simulink model "AMCLIB_TrackObsrv_BAM"  (Simulink 9.3)
settings: Solver=VariableStepAuto  StartTime=0.0  StopTime=10.0  RelTol=1e-3
settings Model: Creator=nxa18952  LastModifiedBy=nxa18952
settings DataIOCC: SaveFormat=Dataset  SignalLoggingSaveFormat=Dataset  ReturnWorkspaceOutputs=on
settings OptimizationCC: LifeSpan=auto
settings DebuggingCC: UnderspecifiedInitializationDetection=Simplified  MergeDetectMultiDrivingBlocksExec=error  FcnCallInpInsideContextMsg=error  SFUnexpectedBacktrackingDiag=error  SFNoUnconditionalDefaultTransitionDiag=error  SFExecutionAtInitializationDiag=warning  ArithmeticOperatorsInVariantConditions=error
settings HardwareCC: ProdBitPerPointer=64  ProdBitPerSizeT=64  ProdBitPerPtrDiffT=64  ProdLargestAtomicFloat=Float  ProdIntDivRoundTo=Zero  ProdEndianess=LittleEndian  ProdWordSize=64  ProdHWDeviceType=Intel->x86-64 (Windows64)
settings ModelReferenceCC: PropagateSignalLabelsOutOfModel=on
settings SFSimCC: SimUseLocalCustomCode=on
settings RTWCC: RTWUseLocalCustomCode=on
settings CodeAppCC: StateflowObjectComments=off
settings GRTTargetCC: TargetLangStandard=C99 (ISO)  CombineOutputUpdateFcns=on  GRTInterface=off
settings ConfigComp: CovMetricSettings=dwe  CovHtmlReporting=off  CovSaveCumulativeToWorkspaceVar=off  CovSaveSingleToWorkspaceVar=off  CovExternalEMLEnable=on

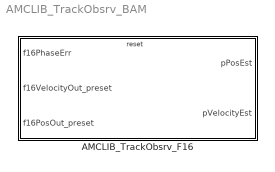
== system AMCLIB_TrackObsrv_BAM ==
  AMCLIB_TrackObsrv_F16 : Subsystem  TreatAsAtomicUnit=on  mask(AMCLIB_TrackObsrv_F16){showStates=Hide (faster execution), resetStatesEnable=Pre-set according to the first set of inputs after reset, f16CC1sc=0, f16CC2sc=0, f16UpperLimit=0, f16LowerLimit=0, u16NShiftPI=0, f16C1=0, u16NShiftI=0}
      mask prompts: showStates "Show internal states"; resetStatesEnable "Internal state after reset"; f16CC1sc "f16CC1sc (GFLIB_ControllerPIrAW - CC1 coefficient)"; f16CC2sc "f16CC2sc (GFLIB_ControllerPIrAW - CC2 coefficient)"; f16UpperLimit "f16UpperLimit (GFLIB_ControllerPIrAW - upper Limit of the controller)"; f16LowerLimit "f16LowerLimit (GFLIB_ControllerPIrAW - lower Limit of the controller)"; u16NShiftPI "u16NShiftPI (GFLIB_ControllerPIrAW - scaling bitwise shift applied to the controller coefficients)"; f16C1 "f16C1 (GFLIB_IntegratorTR - integrator coefficient)"; u16NShiftI "u16NShiftI (GFLIB_IntegratorTR - scaling bitwise shift applied to the integrator coefficient)"
      mask help: Tracking observer in 16-bit fixed-point fractional implementation. This block supports re-initialization of the internal state during simulation. If the block is reset, the outputs of the PI controller and integrator will be aligned with the inputs f16VelocityOut_preset and f16PosOut_preset. Refer to the AMMCLIB User's Guide for further details.
      mask init:
      | if ~evalin('base','exist(''tS8'',''var'')')
      |   if (2 ~= exist('SWLIBS_Typedefs.mat','file'))
      |       error('File SWLIBS_Typedefs.mat is not on the Matlab path. Please add the AMMCLIB "bam" folder in the Matlab Search Path.');
      |   else
      |       evalin('base', 'load(''SWLIBS_Typedefs.mat'')');
      |   end
      | end
      | if showStates == 1
      |     % hidden state variables
      |     if strcmp(get_param([gcb '/f16CC1sc'], 'BlockType'), 'Inport')
      |         posblk = get_param(gcb, 'Position');
      | 
      |         pos = get_param(    [gcb, '/f16CC1sc'], 'Position');
      |         orient = get_param( [gcb, '/f16CC1sc'], 'Orientation');
      |         delete_block(       [gcb, '/f16CC1sc']);
      |         add_block('built-in/Ground', [gcb, '/f16CC1sc'], 'Position', pos, 'Orientation', orient);
      | 
      |         pos = get_param(    [gcb, '/f16CC2sc'], 'Position');
      |         orient = get_param( [gcb, '/f16CC2sc'], 'Orientation');
      |         delete_block(       [gcb, '/f16CC2sc']);
      |         add_block('built-in/Ground', [gcb, '/f16CC2sc'], 'Position', pos, 'Orientation', orient);
      | 
      |         pos = get_param(    [gcb, '/f16UpperLimit'], 'Position');
      |         orient = get_param( [gcb, '/f16UpperLimit'], 'Orientation');
      |         delete_block(       [gcb, '/f16UpperLimit']);
      |         add_block('built-in/Ground', [gcb, '/f16UpperLimit'], 'Position', pos, 'Orientation', orient);
      | 
      |         pos = get_param(    [gcb, '/f16LowerLimit'], 'Position');
      |         orient = get_param( [gcb, '/f16LowerLimit'], 'Orientation');
      |         delete_block(       [gcb, '/f16LowerLimit']);
      |         add_block('built-in/Ground', [gcb, '/f16LowerLimit'], 'Position', pos, 'Orientation', orient);
      | 
      |         pos = get_param(    [gcb, '/u16NShiftPI'], 'Position');
      |         orient = get_param( [gcb, '/u16NShiftPI'], 'Orientation');
      |         delete_block(       [gcb, '/u16NShiftPI']);
      |         add_block('built-in/Ground', [gcb, '/u16NShiftPI'], 'Position', pos, 'Orientation', orient);
      | 
      |         pos = get_param(    [gcb, '/f16C1'], 'Position');
      |         orient = get_param( [gcb, '/f16C1'], 'Orientation');
      |         delete_block(       [gcb, '/f16C1']);
      |         add_block('built-in/Ground', [gcb, '/f16C1'], 'Position', pos, 'Orientation', orient);
      | 
      |         pos = get_param(    [gcb, '/u16NShiftI'], 'Position');
      |         orient = get_param( [gcb, '/u16NShiftI'], 'Orientation');
      |         delete_block(       [gcb, '/u16NShiftI']);
      |         add_block('built-in/Ground', [gcb, '/u16NShiftI'], 'Position', pos, 'Orientation', orient);
      | 
      |         pos = get_param(    [gcb, '/f32Acc'], 'Position');
      |         orient = get_param( [gcb, '/f32Acc'], 'Orientation');
      |         delete_block(       [gcb, '/f32Acc']);
      |         add_block('built-in/Ground', [gcb, '/f32Acc'], 'Position', pos, 'Orientation', orient);
      | 
      |         pos = get_param(    [gcb, '/f16InErrK1'], 'Position');
      |         orient = get_param( [gcb, '/f16InErrK1'], 'Orientation');
      |         delete_block(       [gcb, '/f16InErrK1']);
      |         add_block('built-in/Ground', [gcb, '/f16InErrK1'], 'Position', pos, 'Orientation', orient);
      | 
      |         pos = get_param(    [gcb, '/f32State'], 'Position');
      |         orient = get_param( [gcb, '/f32State'], 'Orientation');
      |         delete_block(       [gcb, '/f32State']);
      |         add_block('built-in/Ground', [gcb, '/f32State'], 'Position', pos, 'Orientation', orient);
      | 
      |         pos = get_param(    [gcb, '/f16InK1'], 'Position');
      |         orient = get_param( [gcb, '/f16InK1'], 'Orientation');
      |         delete_block(       [gcb, '/f16InK1']);
      |         add_block('built-in/Ground', [gcb, '/f16InK1'], 'Position', pos, 'Orientation', orient);
      | 
      | 
      |         pos = get_param(    [gcb '/f32Acc_Out'], 'Position');
      |         orient = get_param( [gcb '/f32Acc_Out'], 'Orientation');
      |         delete_block(       [gcb '/f32Acc_Out']);
      |         add_block('built-in/Terminator', [gcb '/f32Acc_Out'], 'Position', pos, 'Orientation', orient);
      | 
      |         pos = get_param(    [gcb '/f16InErrK1_Out'], 'Position');
      |         orient = get_param( [gcb '/f16InErrK1_Out'], 'Orientation');
      |         delete_block(       [gcb '/f16InErrK1_Out']);
      |         add_block('built-in/Terminator', [gcb '/f16InErrK1_Out'], 'Position', pos, 'Orientation', orient);
      | 
      |         pos = get_param(    [gcb '/f32State_Out'], 'Position');
      |         orient = get_param( [gcb '/f32State_Out'], 'Orientation');
      |         delete_block(       [gcb '/f32State_Out']);
      |         add_block('built-in/Terminator', [gcb '/f32State_Out'], 'Position', pos, 'Orientation', orient);
      | 
      |         pos = get_param(    [gcb '/f16InK1_Out'], 'Position');
      |         orient = get_param( [gcb '/f16InK1_Out'], 'Orientation');
      |         delete_block(       [gcb '/f16InK1_Out']);
      |         add_block('built-in/Terminator', [gcb '/f16InK1_Out'], 'Position', pos, 'Orientation', orient);
      | 
      | 
      |         set_param([gcb '/f16PhaseErr'], 'Port', '1');
      |         set_param([gcb '/f16VelocityOut_preset'], 'Port', '2');
      |         set_param([gcb '/f16PosOut_preset'], 'Port', '3');
      | 
      |         set_param([gcb '/pPosEst'], 'Port', '1');
      |         set_param([gcb '/pVelocityEst'], 'Port', '2');
      | 
      |         set_param(gcb,'MaskEnables',{'on','on','on','on','on','on','on','on','on'});
      | 
      |         if (posblk(4) - posblk(2)) > 100
      |           height = 100;
      |           set_param(gcb,'Position',[posblk(1), posblk(2), posblk(3), posblk(2)+height])
      |         end
      |     end
      | else
      |     % shown state variables
      |     if strcmp(get_param([gcb '/f16CC1sc'], 'BlockType'), 'Ground')
      |         posblk = get_param(gcb, 'Position');
      | 
      |         pos = get_param(    [gcb, '/f16CC1sc'], 'Position');
      |         orient = get_param( [gcb, '/f16CC1sc'], 'Orientation');
      |         delete_block(       [gcb, '/f16CC1sc']);
      |         add_block('built-in/Inport', [gcb, '/f16CC1sc'], 'Position', pos, 'Orientation', orient, 'OutDataTypeStr', 'int16');
      | 
      |         pos = get_param(    [gcb, '/f16CC2sc'], 'Position');
      |         orient = get_param( [gcb, '/f16CC2sc'], 'Orientation');
      |         delete_block(       [gcb, '/f16CC2sc']);
      |         add_block('built-in/Inport', [gcb, '/f16CC2sc'], 'Position', pos, 'Orientation', orient, 'OutDataTypeStr', 'int16');
      | 
      |         pos = get_param(    [gcb, '/f16UpperLimit'], 'Position');
      |         orient = get_param( [gcb, '/f16UpperLimit'], 'Orientation');
      |         delete_block(       [gcb, '/f16UpperLimit']);
      |         add_block('built-in/Inport', [gcb, '/f16UpperLimit'], 'Position', pos, 'Orientation', orient, 'OutDataTypeStr', 'int16');
      | 
      |         pos = get_param(    [gcb, '/f16LowerLimit'], 'Position');
      |         orient = get_param( [gcb, '/f16LowerLimit'], 'Orientation');
      |         delete_block(       [gcb, '/f16LowerLimit']);
      |         add_block('built-in/Inport', [gcb, '/f16LowerLimit'], 'Position', pos, 'Orientation', orient, 'OutDataTypeStr', 'int16');
      | 
      |         pos = get_param(    [gcb, '/u16NShiftPI'], 'Position');
      |         orient = get_param( [gcb, '/u16NShiftPI'], 'Orientation');
      |         delete_block(       [gcb, '/u16NShiftPI']);
      |         add_block('built-in/Inport', [gcb, '/u16NShiftPI'], 'Position', pos, 'Orientation', orient, 'OutDataTypeStr', 'uint16');
      | 
      |         pos = get_param(    [gcb, '/f16C1'], 'Position');
      |         orient = get_param( [gcb, '/f16C1'], 'Orientation');
      |         delete_block(       [gcb, '/f16C1']);
      |         add_block('built-in/Inport', [gcb, '/f16C1'], 'Position', pos, 'Orientation', orient, 'OutDataTypeStr', 'int16');
      | 
      |         pos = get_param(    [gcb, '/u16NShiftI'], 'Position');
      |         orient = get_param( [gcb, '/u16NShiftI'], 'Orientation');
      |         delete_block(       [gcb, '/u16NShiftI']);
      |         add_block('built-in/Inport', [gcb, '/u16NShiftI'], 'Position', pos, 'Orientation', orient, 'OutDataTypeStr', 'uint16');
      | 
      |         pos = get_param(    [gcb, '/f32Acc'], 'Position');
      |         orient = get_param( [gcb, '/f32Acc'], 'Orientation');
      |         delete_block(       [gcb, '/f32Acc']);
      |         add_block('built-in/Inport', [gcb, '/f32Acc'], 'Position', pos, 'Orientation', orient, 'OutDataTypeStr', 'int32');
      | 
      |         pos = get_param(    [gcb, '/f16InErrK1'], 'Position');
      |         orient = get_param( [gcb, '/f16InErrK1'], 'Orientation');
      |         delete_block(       [gcb, '/f16InErrK1']);
      |         add_block('built-in/Inport', [gcb, '/f16InErrK1'], 'Position', pos, 'Orientation', orient, 'OutDataTypeStr', 'int16');
      | 
      |         pos = get_param(    [gcb, '/f32State'], 'Position');
      |         orient = get_param( [gcb, '/f32State'], 'Orientation');
      |         delete_block(       [gcb, '/f32State']);
      |         add_block('built-in/Inport', [gcb, '/f32State'], 'Position', pos, 'Orientation', orient, 'OutDataTypeStr', 'int32');
      | 
      |         pos = get_param(    [gcb, '/f16InK1'], 'Position');
      |         orient = get_param( [gcb, '/f16InK1'], 'Orientation');
      |         delete_block(       [gcb, '/f16InK1']);
      |         add_block('built-in/Inport', [gcb, '/f16InK1'], 'Position', pos, 'Orientation', orient, 'OutDataTypeStr', 'int16');
      | 
      | 
      |         pos = get_param(    [gcb '/f32Acc_Out'], 'Position');
      |         orient = get_param( [gcb '/f32Acc_Out'], 'Orientation');
      |         delete_block(       [gcb '/f32Acc_Out']);
      |         add_block('built-in/Outport', [gcb '/f32Acc_Out'], 'Position', pos, 'Orientation', orient);
      | 
      |         pos = get_param(    [gcb '/f16InErrK1_Out'], 'Position');
      |         orient = get_param( [gcb '/f16InErrK1_Out'], 'Orientation');
      |         delete_block(       [gcb '/f16InErrK1_Out']);
      |         add_block('built-in/Outport', [gcb '/f16InErrK1_Out'], 'Position', pos, 'Orientation', orient);
      | 
      |         pos = get_param(    [gcb '/f32State_Out'], 'Position');
      |         orient = get_param( [gcb '/f32State_Out'], 'Orientation');
      |         delete_block(       [gcb '/f32State_Out']);
      |         add_block('built-in/Outport', [gcb '/f32State_Out'], 'Position', pos, 'Orientation', orient);
      | 
      |         pos = get_param(    [gcb '/f16InK1_Out'], 'Position');
      |         orient = get_param( [gcb '/f16InK1_Out'], 'Orientation');
      |         delete_block(       [gcb '/f16InK1_Out']);
      |         add_block('built-in/Outport', [gcb '/f16InK1_Out'], 'Position', pos, 'Orientation', orient);
      | 
      | 
      |         set_param([gcb '/f16PhaseErr'], 'Port', '1');
      |         set_param([gcb '/f16VelocityOut_preset'], 'Port', '2');
      |         set_param([gcb '/f16PosOut_preset'], 'Port', '3');
      |         set_param([gcb '/f16CC1sc'], 'Port', '4');
      |         set_param([gcb '/f16CC2sc'], 'Port', '5');
      |         set_param([gcb '/f16UpperLimit'], 'Port', '6');
      |         set_param([gcb '/f16LowerLimit'], 'Port', '7');
      |         set_param([gcb '/u16NShiftPI'], 'Port', '8');
      |         set_param([gcb '/f16C1'], 'Port', '9');
      |         set_param([gcb '/u16NShiftI'], 'Port', '10');
      |         set_param([gcb '/f32Acc'], 'Port', '11');
      |         set_param([gcb '/f16InErrK1'], 'Port', '12');
      |         set_param([gcb '/f32State'], 'Port', '13');
      |         set_param([gcb '/f16InK1'], 'Port', '14');
      | 
      |         set_param([gcb '/pPosEst'], 'Port', '1');
      |         set_param([gcb '/pVelocityEst'], 'Port', '2');
      |         set_param([gcb '/f32Acc_Out'], 'Port', '3');
      |         set_param([gcb '/f16InErrK1_Out'], 'Port', '4');
      |         set_param([gcb '/f32State_Out'], 'Port', '5');
      |         set_param([gcb '/f16InK1_Out'], 'Port', '6');
      | 
      |         set_param(gcb,'MaskEnables',{'on','on','off','off','off','off','off','off','off'});
      | 
      |         if (posblk(4) - posblk(2)) < 375
      |           height = 375;
      |           set_param(gcb,'Position',[posblk(1), posblk(2), posblk(3), posblk(2)+height])
      |         end
      |     end
      | end
      settings: RTWSystemCode=Inline
      mask TypeOptions showStates: Hide (faster execution) | Show (allows debugging; connect feedback loops manually)
      mask Callback showStates:
      | maskStr = get_param(gcb,'showStates');
      | if strcmp(maskStr,'Hide (faster execution)'),
      |     set_param(gcb,'MaskEnables',{'on','on','on','on','on','on','on','on','on'});
      | else
      |     set_param(gcb,'MaskEnables',{'on','on','off','off','off','off','off','off','off'});
      | end
      mask TypeOptions resetStatesEnable: Pre-set according to the first set of inputs after reset | Clear to zero
      mask Display:
      | color('black');
      | pos = get_param(gcb, 'Position');
      | width = pos(3) - pos(1);
      | height = pos(4) - pos(2);
      | tX=width/2;
      | tY=height - 25;
      | color('black');
      | text(tX,tY, 'AMCLIB_TrackObsrv_F16', 'horizontalAlignment', 'center');
      | if showStates == 2
      |   color('red');
      |   text(tX,tY - 20, ['debugging mode' char(13) char(10) '(limited performance)'], 'horizontalAlignment', 'center');
      | end

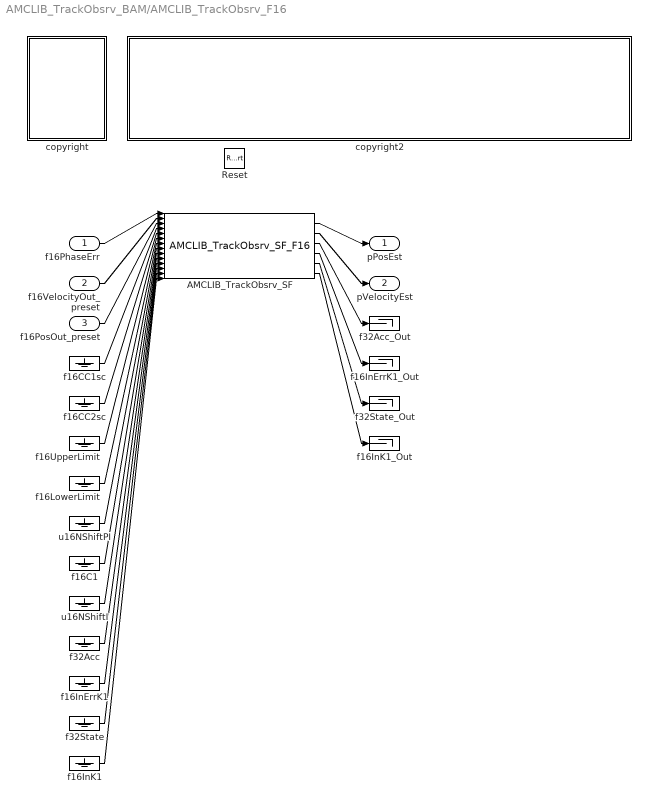
== system AMCLIB_TrackObsrv_BAM/AMCLIB_TrackObsrv_F16 ==
  f16PhaseErr : Inport  OutDataTypeStr=int16
  f16VelocityOut_preset : Inport  Port=2  OutDataTypeStr=int16
  f16PosOut_preset : Inport  Port=3  OutDataTypeStr=int16
  Reset : ResetPort  DisableCoverage=on
  AMCLIB_TrackObsrv_SF : S-Function  FunctionName=AMCLIB_TrackObsrv_SF_F16  Parameters=showStates,resetStatesEnable,f16CC1sc,f16CC2sc,f16UpperLimit,f16LowerLimit,u16NShiftPI,f16C1,u16NShiftI  SFunctionDeploymentMode=off  EnableBusSupport=off
  copyright : Subsystem
      mask Display: text(10,90,'FILE:');text(10,75,'DESRIPTION:');text(10,60,'COPYRIGHT:');text(10,45,'VERSION:');text(10,30,'DATE:')
  copyright2 : Subsystem
      mask Display: text(10,90,'AMCLIB_TrackObsrv_BAM_F16.mdl');text(10,75,'Tracking observer');text(10,60,'NXP 2020');text(10,45,'1.0');text(10,30,'28-Mar-2020');
  f16C1 : Ground
  f16CC1sc : Ground
  f16CC2sc : Ground
  f16InErrK1 : Ground
  f16InErrK1_Out : Terminator
  f16InK1 : Ground
  f16InK1_Out : Terminator
  f16LowerLimit : Ground
  f16UpperLimit : Ground
  f32Acc : Ground
  f32Acc_Out : Terminator
  f32State : Ground
  f32State_Out : Terminator
  u16NShiftI : Ground
  u16NShiftPI : Ground
  pPosEst : Outport
  pVelocityEst : Outport  Port=2
  wires:
  f16PhaseErr/1 -> AMCLIB_TrackObsrv_SF/1
  f16VelocityOut_preset/1 -> AMCLIB_TrackObsrv_SF/2
  f16PosOut_preset/1 -> AMCLIB_TrackObsrv_SF/3
  f16CC1sc/1 -> AMCLIB_TrackObsrv_SF/4
  f16CC2sc/1 -> AMCLIB_TrackObsrv_SF/5
  f16UpperLimit/1 -> AMCLIB_TrackObsrv_SF/6
  f16LowerLimit/1 -> AMCLIB_TrackObsrv_SF/7
  u16NShiftPI/1 -> AMCLIB_TrackObsrv_SF/8
  f16C1/1 -> AMCLIB_TrackObsrv_SF/9
  u16NShiftI/1 -> AMCLIB_TrackObsrv_SF/10
  f32Acc/1 -> AMCLIB_TrackObsrv_SF/11
  f16InErrK1/1 -> AMCLIB_TrackObsrv_SF/12
  f32State/1 -> AMCLIB_TrackObsrv_SF/13
  f16InK1/1 -> AMCLIB_TrackObsrv_SF/14
  AMCLIB_TrackObsrv_SF/1 -> pPosEst/1
  AMCLIB_TrackObsrv_SF/2 -> pVelocityEst/1
  AMCLIB_TrackObsrv_SF/3 -> f32Acc_Out/1
  AMCLIB_TrackObsrv_SF/4 -> f16InErrK1_Out/1
  AMCLIB_TrackObsrv_SF/5 -> f32State_Out/1
  AMCLIB_TrackObsrv_SF/6 -> f16InK1_Out/1

== system AMCLIB_TrackObsrv_BAM/AMCLIB_TrackObsrv_F16/copyright ==

== system AMCLIB_TrackObsrv_BAM/AMCLIB_TrackObsrv_F16/copyright2 ==
